simulink model "pendulum"  (R2020a)
settings: Solver=VariableStepAuto  StartTime=0.0  StopTime=10.0  MaxStep=0.01  RelTol=1e-3
undefined symbols (not defined in the file): g, l
settings Model: Creator=niping1  LastModifiedBy=niping1

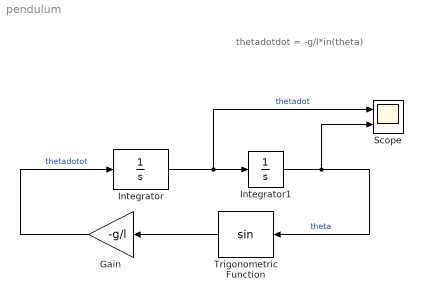
== system pendulum ==
  note: thetadotdot = -g/l*in(theta)
  Gain : Gain  Gain=-g/l
  Integrator : Integrator
  Integrator1 : Integrator  InitialCondition=60
  Scope : Scope  NumInputPorts=2
  Trigonometric Function : Trigonometry
  wires:
  Gain/1 -> Integrator/1  "thetadotot"
  Integrator/1 -> Scope/1, Integrator1/1  "thetadot"
  Integrator1/1 -> Scope/2, Trigonometric Function/1  "theta"
  Trigonometric Function/1 -> Gain/1
